simulink model "Model2_Control"  (R2023b)
settings: Solver=FixedStepAuto  StartTime=0.0  StopTime=Inf  FixedStep=1e-4  RelTol=1e-3
PostLoadFcn:
  | if any(exist('dsrtsu_mdlpostloadfcn', 'file') ~= 0), dsrtsu_mdlpostloadfcn('Execute', bdroot); end
InitFcn:
  | , if any(exist('rtifpga_mdlclblib', 'file') ~= 0), rtifpga_mdlclblib('Init', bdroot); end,
  | , if any(exist('dsmpb_private', 'file') ~= 0), dsmpb_private('dsmpb_mdlclblib', 'Init', bdroot); end,
  | load('LUT_BRUSA_jax_grad.mat')
  | load('daten_nichtlinear_interpoliert.mat')
  | load('Maschinendaten.mat')
  | load('PI_Controller.mat')
  | load('Nonlinear_IPMSM.mat')
values from neighbouring files (symbols this model uses):
  p = 3    [Maschinendaten.mat]    (also in Maschinendaten_Vorgabe.m; Messdaten_Interpoliert.m; test_ModelParameters.m = evalin('base', 'p'))
undefined symbols (not defined in the file or in its folder): T_L, T_svm, U_DC
libraries: dsmpblib x8, electric_drives_and_control_components_library x7
PreSaveFcn:
  | , if any(exist('dsmpb_private', 'file') ~= 0), dsmpb_private('dsmpb_mdlclblib', 'PreSave', bdroot); end,
CloseFcn:
  | , if any(exist('dsmpb_private', 'file') ~= 0), dsmpb_private('dsmpb_mdlclblib', 'Close', bdroot); end,
settings Model: DSRTSU_INTERNAL_RTIFPGA=210  DSRTSU_INTERNAL_RTISTBM_VER=24.2  DSMPB_ID_DATA={'111',struct('BlockId','f4f53aad-8f82-48e8-b261-2ca4efd95365403','SignalIds',{{'f4f53aad-8f82-48e8-b261-2ca4efd95365403_1'}}),'112',struct('BlockId','f4f53aad-8f82-48e8-b261-2ca4efd95365404','SignalIds',{{'f4f53aad-8f82-48e8-b261-2ca4efd95365404_1'}}),'115',struct('BlockId','7ea6da62-da15-4185-95a6-74a1fe28ce7c','SignalIds',{{'cd385c15-7a5d-4812-9b24-23e45cac895a'}}),'116',struct('BlockId','05e47a6e-34ef-4aed-aa2e-c2081137d83f','SignalIds',{{'11cd64ab-ca30-49e8-be0b-0ddcef0800fc'}}),'118',struct('BlockId','6229b99e-c717-4f87-9340-18379a515b71','SignalIds',{{'a711d870-74e6-46e3-a328-b62934671b6c'}}),'120',struct('BlockId','91a71344-0d5d-41ea-b6f7-e376cbcf0b1a','SignalIds',{{'402d4722-ce2f-45a1-8201-9d5d2edb07c0'}}),'6',struct('BlockId','e93b0527-b478-40ef-84bc-d29f8830316f','SignalIds',{{'daf77724-8c5c-420c-be4a-0b473ed67fee'}}),'7',struct('BlockId','05602117-b862-48e4-b8a5-fd288bdfb97b','SignalIds',{{'e086e407-aa55-4b5c-bf12-996f5d931d03'}})}  Creator=Student  LastModifiedBy=Student
settings OptimizationCC: BlockReduction=off  ConditionallyExecuteInputs=off  OptimizeBlockIOStorage=off  BufferReuse=off
settings DebuggingCC: TasksWithSamePriorityMsg=none
settings HardwareCC: ProdBitPerLong=64  ProdLargestAtomicInteger=Integer  ProdWordSize=32  ProdLongLongMode=on  ProdHWDeviceType=Custom Processor->Custom
settings ModelReferenceCC: EnableParallelModelReferenceBuilds=on
settings RTWCC: Description=dSPACE Target DSRT - Generates SIC files for import by ConfigurationDesk and VEOS. Provides code generation for Simulink models imported in ConfigurationDesk.  SystemTargetFile=dsrt.tlc  GenCodeOnly=on  MakeCommand=make_dsrt  TemplateMakefile=dsrt_default_tmf  RTWVerbose=off
settings STFCustomTargetCC: ParMdlRefBuildCompliant=on  SystemTargetFile=dsrt.tlc
settings GRTTargetCC: CompOptLevelCompliant=off  ConcurrentExecutionCompliant=off  CombineOutputUpdateFcns=off  MatFileLogging=off  CPPClassGenCompliant=off  UseToolchainInfoCompliant=off

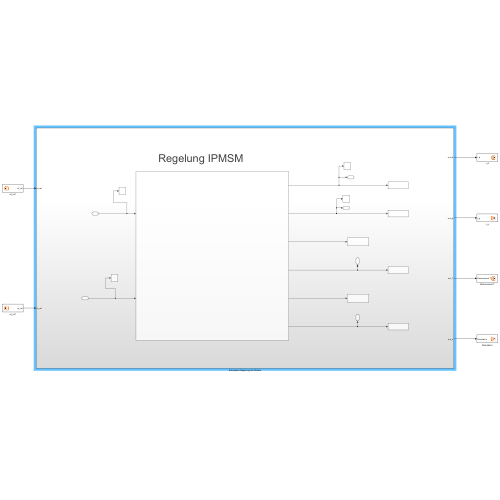
[thumbnail: Simulink's stored preview of the top-level diagram]
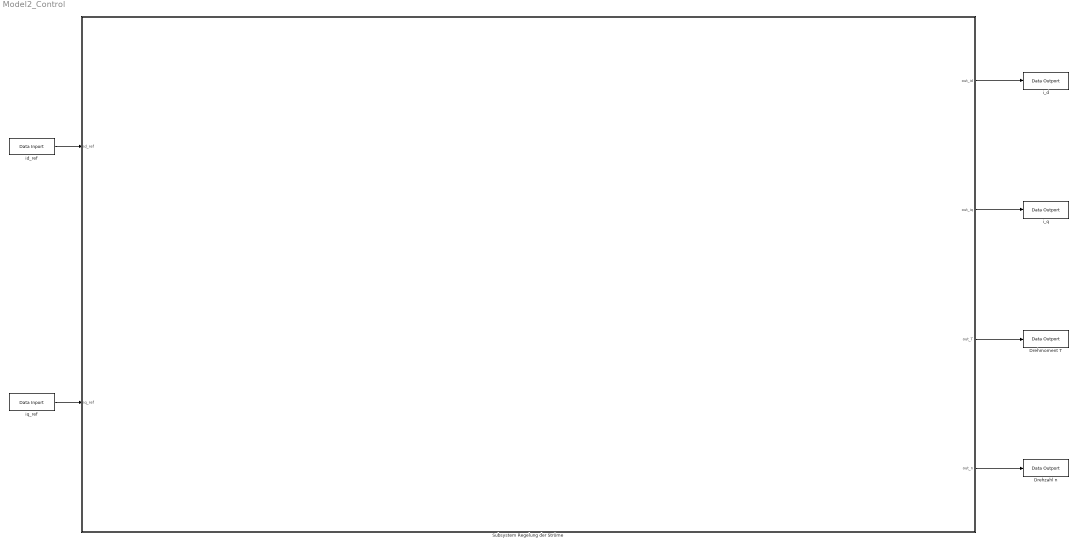
== system Model2_Control ==
  Drehmoment T : dsmpblib/Data Outport  Priority=-10000
      settings: SourceProductName=dSPACE Model Interface Package for Simulink (MIPS)
  Drehzahl n : dsmpblib/Data Outport  Priority=-10000
      settings: SourceProductName=dSPACE Model Interface Package for Simulink (MIPS)
  Subsystem Regelung der Ströme : Subsystem
  i_d : dsmpblib/Data Outport  Priority=-10000
      settings: SourceProductName=dSPACE Model Interface Package for Simulink (MIPS)
  i_q : dsmpblib/Data Outport  Priority=-10000
      settings: SourceProductName=dSPACE Model Interface Package for Simulink (MIPS)
  id_ref : dsmpblib/Data Inport  Priority=10000
      settings: SourceProductName=dSPACE Model Interface Package for Simulink (MIPS)
  iq_ref : dsmpblib/Data Inport  Priority=10000
      settings: SourceProductName=dSPACE Model Interface Package for Simulink (MIPS)
  wires:
  id_ref/1 -> Subsystem Regelung der Ströme/1(id_ref)
  iq_ref/1 -> Subsystem Regelung der Ströme/2(iq_ref)
  Subsystem Regelung der Ströme/1(out_id) -> i_d/1
  Subsystem Regelung der Ströme/2(out_iq) -> i_q/1
  Subsystem Regelung der Ströme/3(out_T) -> Drehmoment T/1
  Subsystem Regelung der Ströme/4(out_n) -> Drehzahl n/1

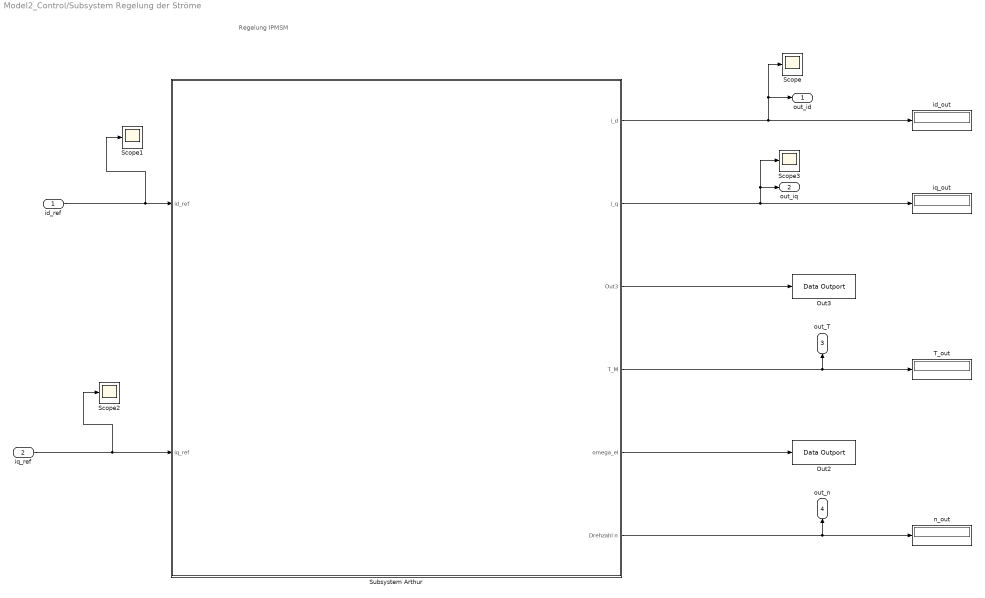
== system Model2_Control/Subsystem Regelung der Ströme ==
  note: Regelung IPMSM
  id_ref : Inport
  iq_ref : Inport  Port=2
  Out2 : dsmpblib/Data Outport  Priority=-10000
      settings: SourceProductName=dSPACE Model Interface Package for Simulink (MIPS)
  Out3 : dsmpblib/Data Outport  Priority=-10000
      settings: SourceProductName=dSPACE Model Interface Package for Simulink (MIPS)
  Scope{,1..3} (4 alike) : Scope
  Subsystem Arthur : Subsystem
  T_out : Display
  id_out : Display
  iq_out : Display
  n_out : Display
  out_id : Outport
  out_iq : Outport  Port=2
  out_T : Outport  Port=3
  out_n : Outport  Port=4
  wires:
  Subsystem Arthur/3(Out3) -> Out3/1
  Subsystem Arthur/5(omega_el) -> Out2/1
  Subsystem Arthur/4(T_M) -> T_out/1, out_T/1
  Subsystem Arthur/1(i_d) -> id_out/1, Scope/1, out_id/1
  id_ref/1 -> Subsystem Arthur/1(id_ref), Scope1/1
  Subsystem Arthur/6(Drehzahl n) -> n_out/1, out_n/1
  Subsystem Arthur/2(i_q) -> iq_out/1, Scope3/1, out_iq/1
  iq_ref/1 -> Subsystem Arthur/2(iq_ref), Scope2/1

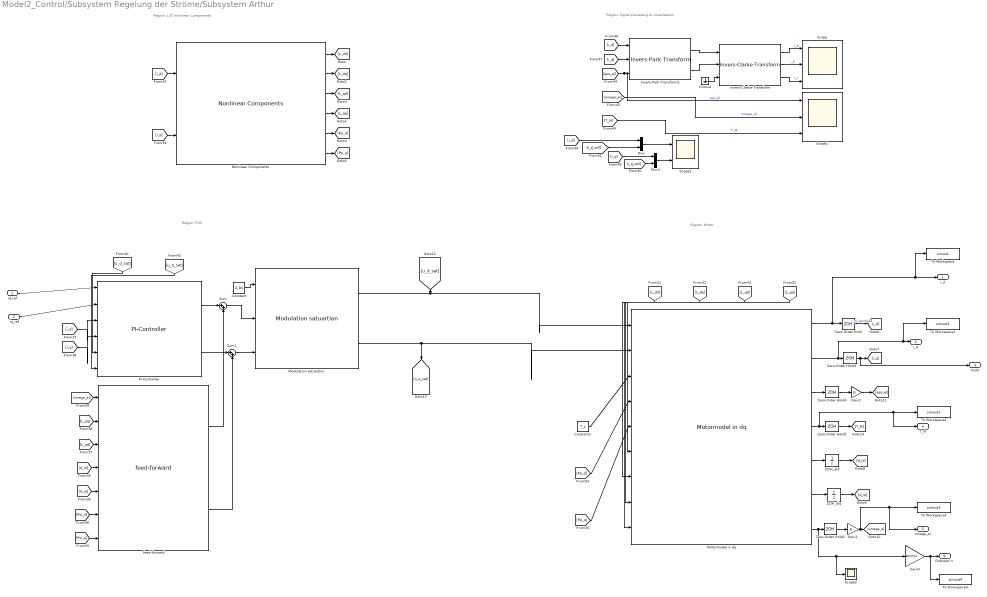
== system Model2_Control/Subsystem Regelung der Ströme/Subsystem Arthur ==
  note: Region: Motor
  note: Region: FOC
  note: Region: LUT nonlinear Components
  note: Region: Signal processing & visualization
  id_ref : Inport
  iq_ref : Inport  Port=2
  Constant : Constant  Value=U_DC
  Constant1 : Constant  Value=T_L
  Gain1 : Gain  Gain=p
  Gain2 : Gain  Gain=p
  Gain3 : Gain  Gain=60/(2*pi)
  Ground : Ground
  Invers-Clarke-Transform : electric_drives_and_control_components_library/Transformation matrices/Invers-Clarke-Transform
  Invers-Park-Transform1 : electric_drives_and_control_components_library/Transformation matrices/Invers-Park-Transform
  Modulation satuartion : electric_drives_and_control_components_library/Controller & observer algorithms/FOC/Modulation Satuartion/Modulation satuartion
  Motormodel in dq : electric_drives_and_control_components_library/Electric Drive Models/PMSM/Motormodel in dq  Parameter2=T_N  Parameter1=R_s  Parameter3=Psi_p  Parameter4=p  Parameter5=omega_M_0  Parameter6=J  Parameter7=eps_M_0  Parameter8=L_dd  Parameter9=L_dq  Parameter10=L_qd  Parameter11=L_qq
  Mux : Mux  Inputs=2
  Mux1 : Mux  Inputs=2
  Nonlinear Components : electric_drives_and_control_components_library/Nonlinear & linear components IPMSM/Nonlinear Components  Parameter6=L_dd  Parameter4=L_dq  Parameter5=L_qd  Parameter1=L_qq  Parameter2=Psi_d  Parameter3=Psi_q
  PI-Controller : electric_drives_and_control_components_library/Controller & observer algorithms/FOC/Controller/PI-Controller  Parameter6=KP_d  Parameter1=KI_d  Parameter2=KP_q  Parameter3=KI_q  Parameter4=awu
  Scope : Scope  NumInputPorts=3
  Scope1 : Scope  NumInputPorts=3
  Scope2 : Scope  NumInputPorts=2
  Scope3 : Scope
  Sum : Sum  Inputs=|++
  Sum1 : Sum  Inputs=|++
  To Workspace : ToWorkspace  VariableName=simout  SaveFormat=Timeseries  SampleTime=-1
  To Workspace1 : ToWorkspace  VariableName=simout1  SaveFormat=Timeseries  SampleTime=-1
  To Workspace2 : ToWorkspace  VariableName=simout2  SaveFormat=Timeseries  SampleTime=-1
  To Workspace3 : ToWorkspace  VariableName=simout3  SaveFormat=Timeseries  SampleTime=-1
  To Workspace4 : ToWorkspace  VariableName=simout4  SaveFormat=Timeseries  SampleTime=-1
  ZOH_did : UnitDelay  SampleTime=-1  HasFrameUpgradeWarning=on
  ZOH_diq : UnitDelay  SampleTime=-1  HasFrameUpgradeWarning=on
  Zero-Order Hold{,2..5} (5 alike) : ZeroOrderHold  SampleTime=T_svm
  feed-forward : electric_drives_and_control_components_library/Controller & observer algorithms/FOC/feed-forward/feed-forward  Parameter1=Psi_p  Parameter2=L_dd  Parameter3=L_dq  Parameter4=L_qd  Parameter5=L_qq
  i_d : Outport
  i_q : Outport  Port=2
  Out3 : Outport  Port=3
  T_M : Outport  Port=4
  omega_el : Outport  Port=5
  Drehzahl n : Outport  Port=6
  wires:
  Gain3/1 -> Drehzahl n/1, To Workspace4/1
  Motormodel in dq/6 -> ZOH_diq/1
  PI-Controller/1 -> Sum/1
  Motormodel in dq/1 -> i_d/1, To Workspace/1, Zero-Order Hold/1
  [i_q] -> Invers-Park-Transform1/2
  Zero-Order Hold4/1 -> Gain2/1
  Nonlinear Components/1 -> [L_dd]
  Motormodel in dq/5 -> ZOH_did/1
  [L_dd] -> Motormodel in dq/6
  feed-forward/1 -> Sum/2
  Sum1/1 -> Modulation satuartion/3
  [L_qd] -> feed-forward/3
  [i_d_soll] -> Mux/2
  [i_q_soll] -> Mux1/2
  [u_d_sat] -> PI-Controller/5
  [omega_el] -> Scope1/2  "omega_el"
  Modulation satuartion/1 -> Motormodel in dq/1, [u_d_sat]
  Zero-Order Hold2/1 -> Gain1/1
  feed-forward/2 -> Sum1/2
  Gain1/1 -> [omega_el], To Workspace3/1, omega_el/1
  Nonlinear Components/6 -> [Psi_q]
  Motormodel in dq/7 -> Zero-Order Hold2/1, Scope3/1, Gain3/1
  [i_d] -> Nonlinear Components/1
  [Psi_d] -> Motormodel in dq/4
  [omega_el] -> feed-forward/1
  [L_qd] -> Motormodel in dq/8
  Invers-Clarke-Transform/2 -> Scope/2  "i_b"
  Gain2/1 -> [eps_el]
  Modulation satuartion/2 -> Motormodel in dq/2, [u_q_sat]
  ZOH_diq/1 -> [d_iq]
  [i_d] -> Invers-Park-Transform1/1
  Invers-Clarke-Transform/3 -> Scope/3  "i_c"
  [eps_el] -> Scope1/1, Invers-Park-Transform1/3  "eps_el"
  Constant/1 -> Modulation satuartion/1
  Ground/1 -> Invers-Clarke-Transform/3
  Nonlinear Components/2 -> [L_dq]
  Mux/1 -> Scope2/1
  [i_q] -> Mux1/1
  [i_q] -> Nonlinear Components/2
  ZOH_did/1 -> [d_id]
  [L_qq] -> Motormodel in dq/9
  [Psi_q] -> Motormodel in dq/5
  [Psi_q] -> feed-forward/7
  Invers-Clarke-Transform/1 -> Scope/1  "i_a"
  [T_M] -> Scope1/3  "T_M"
  Constant1/1 -> Motormodel in dq/3
  Mux1/1 -> Scope2/2
  [i_d] -> Mux/1
  Zero-Order Hold5/1 -> [T_M]
  Nonlinear Components/3 -> [L_qd]
  [i_q] -> PI-Controller/4
  PI-Controller/2 -> Sum1/1
  Nonlinear Components/4 -> [L_qq]
  Zero-Order Hold3/1 -> Out3/1, [i_q]
  Sum/1 -> Modulation satuartion/2
  Zero-Order Hold/1 -> [i_d]  "i_d_sampled"
  Invers-Park-Transform1/2 -> Invers-Clarke-Transform/2
  Motormodel in dq/4 -> Zero-Order Hold5/1, T_M/1, To Workspace2/1
  [L_dq] -> Motormodel in dq/7
  [d_iq] -> feed-forward/5
  [i_d] -> PI-Controller/3
  Invers-Park-Transform1/1 -> Invers-Clarke-Transform/1
  [u_q_sat] -> PI-Controller/6
  Motormodel in dq/3 -> Zero-Order Hold4/1
  Motormodel in dq/2 -> i_q/1, To Workspace1/1, Zero-Order Hold3/1
  Nonlinear Components/5 -> [Psi_d]
  [Psi_d] -> feed-forward/6
  [d_id] -> feed-forward/4
  iq_ref/1 -> PI-Controller/2
  [L_dq] -> feed-forward/2
  id_ref/1 -> PI-Controller/1
